simulink model "ldr"  (R2022b)
settings: Solver=VariableStepAuto  StartTime=0.0  StopTime=10.0  RelTol=1e-3
settings Model: Creator=shadr  LastModifiedBy=marak

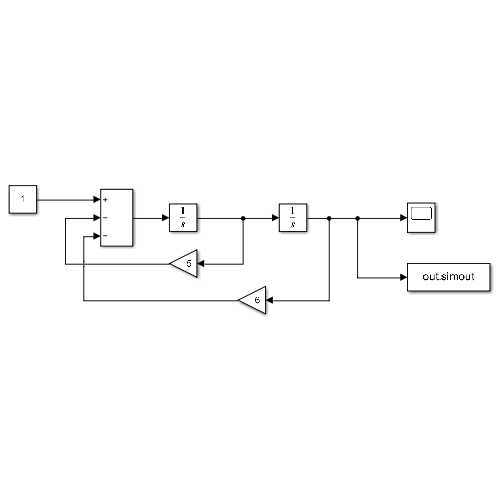
[thumbnail: Simulink's stored preview of the top-level diagram]
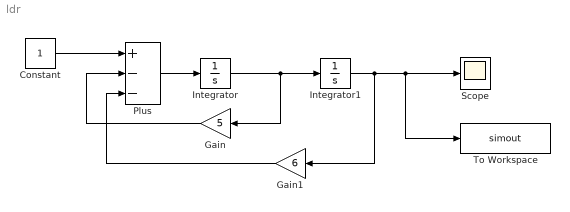
== system ldr ==
  Constant : Constant
  Gain : Gain  Gain=5
  Gain1 : Gain  Gain=6
  Integrator : Integrator
  Integrator1 : Integrator
  Plus : Sum  Inputs=+--
  Scope : Scope
  To Workspace : ToWorkspace  VariableName=simout  SaveFormat=Timeseries  SampleTime=-1
  wires:
  Integrator/1 -> Gain/1, Integrator1/1
  Constant/1 -> Plus/1
  Gain/1 -> Plus/2
  Plus/1 -> Integrator/1
  Integrator1/1 -> Gain1/1, To Workspace/1, Scope/1
  Gain1/1 -> Plus/3
